simulink model "torqueWalking"  (Simulink 8.8)
settings: Solver=FixedStepDiscrete  StartTime=0.0  StopTime=Config.t_end  FixedStep=Config.t_step  RelTol=1e-3  EnableMultiTasking=on
InitFcn:
  | cd(fileparts(which(bdroot)));
  | initTorqueWalking;
undefined symbols (not defined in the file or in its folder): biasVectorConstraint_feet, Config, ConstraintMatrix_feet, DiscIntNeverNeededParam, Gains, ROBOT_DOF, Sat
libraries: WBToolboxLibrary x98
(part 2 of 3)

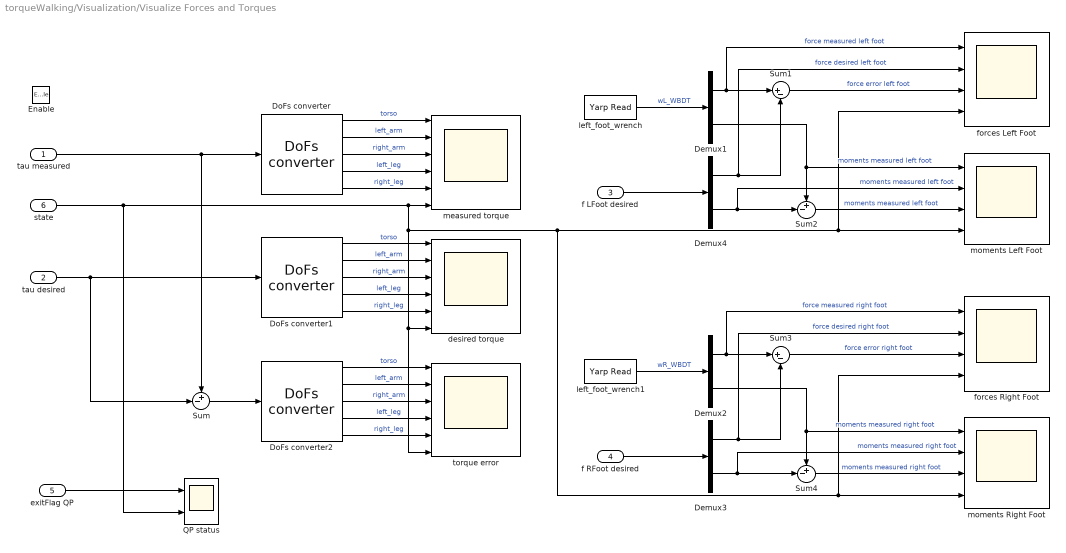
== system torqueWalking/Visualization/Visualize Forces and Torques ==
  tau measured : Inport
  tau desired : Inport  Port=2
  f LFoot desired : Inport  Port=3
  f RFoot desired : Inport  Port=4
  exitFlag QP : Inport  Port=5
  state : Inport  Port=6
  Enable : EnablePort
  Demux{1..4} (4 alike) : Demux  Outputs=[3;3]
  DoFs converter : WBToolboxLibrary/Utilities/DoFs converter  yarp2WBIOption=From WBI to YARP  robotName=WBT_robotName  localName=WBT_modelName  wbiFile=WBT_wbiFilename  wbiList=WBT_wbiList
  DoFs converter1 : WBToolboxLibrary/Utilities/DoFs converter  yarp2WBIOption=From WBI to YARP  robotName=WBT_robotName  localName=WBT_modelName  wbiFile=WBT_wbiFilename  wbiList=WBT_wbiList
  DoFs converter2 : WBToolboxLibrary/Utilities/DoFs converter  yarp2WBIOption=From WBI to YARP  robotName=WBT_robotName  localName=WBT_modelName  wbiFile=WBT_wbiFilename  wbiList=WBT_wbiList
  QP status : Scope  NumInputPorts=2
  Sum : Sum  Inputs=+-|
  Sum1 : Sum  Inputs=|+-
  Sum2 : Sum  Inputs=+-|
  Sum3 : Sum  Inputs=|+-
  Sum4 : Sum  Inputs=+-|
  desired torque : Scope  NumInputPorts=6
  forces Left Foot : Scope  NumInputPorts=4
  forces Right Foot : Scope  NumInputPorts=4
  left_foot_wrench : WBToolboxLibrary/Utilities/Yarp Read  portName=Ports.LEFT_FOOT_EXT_WRENCH  signalSize=6  blocking=off  timestamp=off  autoconnect=on  errorOnConnection=on
  left_foot_wrench1 : WBToolboxLibrary/Utilities/Yarp Read  portName=Ports.LEFT_FOOT_EXT_WRENCH  signalSize=6  blocking=off  timestamp=off  autoconnect=on  errorOnConnection=on
  measured torque : Scope  NumInputPorts=6
  moments Left Foot : Scope  NumInputPorts=4
  moments Right Foot : Scope  NumInputPorts=4
  torque error : Scope  NumInputPorts=6
  wires:
  Sum2/1 -> moments Left Foot/3  "moments measured left foot"
  state/1 -> QP status/2, torque error/6, desired torque/6, forces Right Foot/4, moments Right Foot/4, forces Left Foot/4, moments Left Foot/4, measured torque/6
  DoFs converter1/2 -> desired torque/2  "left_arm"
  Demux4/1 -> forces Left Foot/2, Sum1/2  "force desired left foot"
  DoFs converter2/1 -> torque error/1  "torso"
  DoFs converter1/4 -> desired torque/4  "left_leg"
  Demux4/2 -> moments Left Foot/2, Sum2/2  "moments measured left foot"
  DoFs converter/1 -> measured torque/1  "torso"
  DoFs converter2/3 -> torque error/3  "right_arm"
  f RFoot desired/1 -> Demux3/1
  DoFs converter1/1 -> desired torque/1  "torso"
  Sum4/1 -> moments Right Foot/3  "moments measured right foot"
  tau desired/1 -> Sum/2, DoFs converter1/1
  Demux2/1 -> forces Right Foot/1, Sum3/1  "force measured right foot"
  DoFs converter2/2 -> torque error/2  "left_arm"
  Sum3/1 -> forces Right Foot/3  "force error right foot"
  DoFs converter/5 -> measured torque/5  "right_leg"
  DoFs converter2/5 -> torque error/5  "right_leg"
  exitFlag QP/1 -> QP status/1
  left_foot_wrench/1 -> Demux1/1  "wL_WBDT"
  DoFs converter1/3 -> desired torque/3  "right_arm"
  Demux3/1 -> forces Right Foot/2, Sum3/2  "force desired right foot"
  f LFoot desired/1 -> Demux4/1
  Sum1/1 -> forces Left Foot/3  "force error left foot"
  tau measured/1 -> Sum/1, DoFs converter/1
  DoFs converter1/5 -> desired torque/5  "right_leg"
  DoFs converter/2 -> measured torque/2  "left_arm"
  DoFs converter/3 -> measured torque/3  "right_arm"
  Demux3/2 -> moments Right Foot/2, Sum4/2  "moments measured right foot"
  Sum/1 -> DoFs converter2/1
  Demux1/1 -> forces Left Foot/1, Sum1/1  "force measured left foot"
  DoFs converter/4 -> measured torque/4  "left_leg"
  Demux1/2 -> moments Left Foot/1, Sum2/1  "moments measured left foot"
  left_foot_wrench1/1 -> Demux2/1  "wR_WBDT"
  DoFs converter2/4 -> torque error/4  "left_leg"
  Demux2/2 -> moments Right Foot/1, Sum4/1  "moments measured right foot"

== system torqueWalking/Visualization/Visualize Gain Scheduling ==
  Kp_CoM : Inport
  Kd_CoM : Inport  Port=2
  Kp_LFoot : Inport  Port=3
  Kd_LFoot : Inport  Port=4
  Kp_RFoot : Inport  Port=5
  Kd_RFoot : Inport  Port=6
  Kp_rot_task : Inport  Port=7
  Kd_rot_task : Inport  Port=8
  impedances : Inport  Port=9
  dampings : Inport  Port=10
  state : Inport  Port=11
  Enable : EnablePort
  DoFs converter1 : WBToolboxLibrary/Utilities/DoFs converter  yarp2WBIOption=From WBI to YARP  robotName=WBT_robotName  localName=WBT_modelName  wbiFile=WBT_wbiFilename  wbiList=WBT_wbiList
  DoFs converter4 : WBToolboxLibrary/Utilities/DoFs converter  yarp2WBIOption=From WBI to YARP  robotName=WBT_robotName  localName=WBT_modelName  wbiFile=WBT_wbiFilename  wbiList=WBT_wbiList
  joint position gains : Scope  NumInputPorts=6
  joint valocity gains : Scope  NumInputPorts=6
  pos gains CoM : Scope  NumInputPorts=2
  pos gains LFoot : Scope  NumInputPorts=2
  pos gains RFoot : Scope  NumInputPorts=2
  pos gains rot task : Scope  NumInputPorts=2
  vel gains CoM : Scope  NumInputPorts=2
  vel gains LFoot : Scope  NumInputPorts=2
  vel gains RFoot : Scope  NumInputPorts=2
  vel gains rot task : Scope  NumInputPorts=2
  wires:
  Kp_CoM/1 -> pos gains CoM/1
  Kp_LFoot/1 -> pos gains LFoot/1
  Kp_RFoot/1 -> pos gains RFoot/1
  Kp_rot_task/1 -> pos gains rot task/1
  state/1 -> vel gains LFoot/2, pos gains LFoot/2, vel gains CoM/2, vel gains rot task/2, pos gains rot task/2, vel gains RFoot/2, joint valocity gains/6, joint position gains/6, pos gains RFoot/2, pos gains CoM/2
  Kd_CoM/1 -> vel gains CoM/1
  Kd_LFoot/1 -> vel gains LFoot/1
  Kd_RFoot/1 -> vel gains RFoot/1
  Kd_rot_task/1 -> vel gains rot task/1
  DoFs converter4/2 -> joint position gains/2  "left_arm"
  DoFs converter4/1 -> joint position gains/1  "torso"
  DoFs converter4/4 -> joint position gains/4  "left_leg"
  DoFs converter4/3 -> joint position gains/3  "right_arm"
  DoFs converter4/5 -> joint position gains/5  "right_leg"
  DoFs converter1/2 -> joint valocity gains/2  "left_arm"
  DoFs converter1/1 -> joint valocity gains/1  "torso"
  DoFs converter1/4 -> joint valocity gains/4  "left_leg"
  DoFs converter1/3 -> joint valocity gains/3  "right_arm"
  DoFs converter1/5 -> joint valocity gains/5  "right_leg"
  impedances/1 -> DoFs converter4/1
  dampings/1 -> DoFs converter1/1

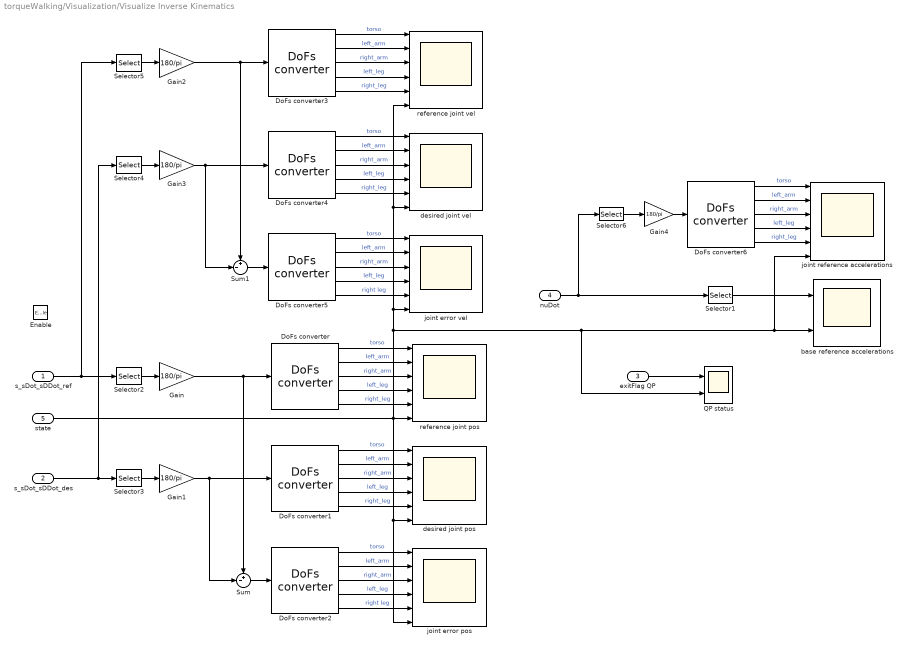
== system torqueWalking/Visualization/Visualize Inverse Kinematics ==
  s_sDot_sDDot_ref : Inport
  s_sDot_sDDot_des : Inport  Port=2
  exitFlag QP : Inport  Port=3
  nuDot : Inport  Port=4
  state : Inport  Port=5
  Enable : EnablePort
  DoFs converter{,1..6} (7 alike) : WBToolboxLibrary/Utilities/DoFs converter  yarp2WBIOption=From WBI to YARP  robotName=WBT_robotName  localName=WBT_modelName  wbiFile=WBT_wbiFilename  wbiList=WBT_wbiList
  Gain{,1..4} (5 alike) : Gain  Gain=180/pi
  QP status : Scope  NumInputPorts=2
  Selector1 : Selector  InputPortWidth=ROBOT_DOF+6  IndexOptions=Index vector (dialog)  Indices=[1:6]  OutputSizes=1
  Selector2 : Selector  NumberOfDimensions=2  InputPortWidth=ROBOT_DOF  IndexOptions=Index vector (dialog),Index vector (dialog)  Indices=[1:ROBOT_DOF],1  OutputSizes=1,1
  Selector3 : Selector  NumberOfDimensions=2  InputPortWidth=ROBOT_DOF  IndexOptions=Index vector (dialog),Index vector (dialog)  Indices=[1:ROBOT_DOF],1  OutputSizes=1,1
  Selector4 : Selector  NumberOfDimensions=2  InputPortWidth=ROBOT_DOF  IndexOptions=Index vector (dialog),Index vector (dialog)  Indices=[1:ROBOT_DOF],2  OutputSizes=1,1
  Selector5 : Selector  NumberOfDimensions=2  InputPortWidth=ROBOT_DOF  IndexOptions=Index vector (dialog),Index vector (dialog)  Indices=[1:ROBOT_DOF],2  OutputSizes=1,1
  Selector6 : Selector  InputPortWidth=ROBOT_DOF+6  IndexOptions=Index vector (dialog)  Indices=[7:ROBOT_DOF+6]  OutputSizes=1
  Sum : Sum  Inputs=+-|
  Sum1 : Sum  Inputs=+-|
  base reference accelerations : Scope  NumInputPorts=2
  desired joint pos : Scope  NumInputPorts=6
  desired joint vel : Scope  NumInputPorts=6
  joint error pos : Scope  NumInputPorts=6
  joint error vel : Scope  NumInputPorts=6
  joint reference accelerations : Scope  NumInputPorts=6
  reference joint pos : Scope  NumInputPorts=6
  reference joint vel : Scope  NumInputPorts=6
  wires:
  DoFs converter1/2 -> desired joint pos/2  "left_arm"
  DoFs converter/5 -> reference joint pos/5  "right_leg"
  DoFs converter2/1 -> joint error pos/1  "torso"
  DoFs converter/4 -> reference joint pos/4  "left_leg"
  DoFs converter/2 -> reference joint pos/2  "left_arm"
  DoFs converter1/1 -> desired joint pos/1  "torso"
  DoFs converter1/4 -> desired joint pos/4  "left_leg"
  DoFs converter1/3 -> desired joint pos/3  "right_arm"
  DoFs converter/3 -> reference joint pos/3  "right_arm"
  DoFs converter2/2 -> joint error pos/2  "left_arm"
  DoFs converter/1 -> reference joint pos/1  "torso"
  DoFs converter1/5 -> desired joint pos/5  "right_leg"
  DoFs converter2/4 -> joint error pos/4  "left_leg"
  Sum/1 -> DoFs converter2/1
  DoFs converter2/3 -> joint error pos/3  "right_arm"
  Gain/1 -> Sum/1, DoFs converter/1
  Gain1/1 -> Sum/2, DoFs converter1/1
  DoFs converter4/2 -> desired joint vel/2  "left_arm"
  DoFs converter3/5 -> reference joint vel/5  "right_leg"
  DoFs converter5/1 -> joint error vel/1  "torso"
  DoFs converter3/4 -> reference joint vel/4  "left_leg"
  DoFs converter3/2 -> reference joint vel/2  "left_arm"
  s_sDot_sDDot_ref/1 -> Selector5/1, Selector2/1
  DoFs converter4/1 -> desired joint vel/1  "torso"
  DoFs converter4/4 -> desired joint vel/4  "left_leg"
  DoFs converter4/3 -> desired joint vel/3  "right_arm"
  DoFs converter3/3 -> reference joint vel/3  "right_arm"
  DoFs converter5/2 -> joint error vel/2  "left_arm"
  DoFs converter3/1 -> reference joint vel/1  "torso"
  s_sDot_sDDot_des/1 -> Selector4/1, Selector3/1
  DoFs converter4/5 -> desired joint vel/5  "right_leg"
  DoFs converter5/4 -> joint error vel/4  "left_leg"
  Sum1/1 -> DoFs converter5/1
  DoFs converter5/3 -> joint error vel/3  "right_arm"
  Gain2/1 -> Sum1/1, DoFs converter3/1
  Gain3/1 -> Sum1/2, DoFs converter4/1
  DoFs converter5/5 -> joint error vel/5  "right leg"
  DoFs converter2/5 -> joint error pos/5  "right leg"
  Selector1/1 -> base reference accelerations/1
  Selector2/1 -> Gain/1
  Selector3/1 -> Gain1/1
  Selector4/1 -> Gain3/1
  Selector5/1 -> Gain2/1
  DoFs converter6/5 -> joint reference accelerations/5  "right_leg"
  DoFs converter6/1 -> joint reference accelerations/1  "torso"
  DoFs converter6/4 -> joint reference accelerations/4  "left_leg"
  DoFs converter6/3 -> joint reference accelerations/3  "right_arm"
  DoFs converter6/2 -> joint reference accelerations/2  "left_arm"
  nuDot/1 -> Selector6/1, Selector1/1
  Gain4/1 -> DoFs converter6/1
  Selector6/1 -> Gain4/1
  state/1 -> reference joint vel/6, desired joint vel/6, joint error vel/6, QP status/2, joint reference accelerations/6, base reference accelerations/2, joint error pos/6, desired joint pos/6, reference joint pos/6
  exitFlag QP/1 -> QP status/1

== system torqueWalking/Visualization/Visualize Robot State ==
  s : Inport
  w_H_b : Inport  Port=2
  nu : Inport  Port=3
  state : Inport  Port=4
  s_des : Inport  Port=5
  feetInContact : Inport  Port=6
  Enable : EnablePort
  DoFs converter{,1..3} (4 alike) : WBToolboxLibrary/Utilities/DoFs converter  yarp2WBIOption=From WBI to YARP  robotName=WBT_robotName  localName=WBT_modelName  wbiFile=WBT_wbiFilename  wbiList=WBT_wbiList
  Gain : Gain  Gain=180/pi
  Gain1 : Gain  Gain=180/pi
  Gain2 : Gain  Gain=180/pi
  Selector : Selector  NumberOfDimensions=2  InputPortWidth=3  IndexOptions=Index vector (dialog),Index vector (dialog)  Indices=[1:3],4  OutputSizes=1,1
  Selector1 : Selector  InputPortWidth=ROBOT_DOF+6  IndexOptions=Index vector (dialog)  Indices=[1:6]  OutputSizes=1
  Selector2 : Selector  InputPortWidth=ROBOT_DOF+6  IndexOptions=Index vector (dialog)  Indices=[7:ROBOT_DOF+6]  OutputSizes=1
  Sum : Sum  Inputs=+-|
  base position : Scope  NumInputPorts=2
  base velocity : Scope  NumInputPorts=2
  desired joint pos : Scope  NumInputPorts=6
  feet in contact : Scope  NumInputPorts=2
  joint error : Scope  NumInputPorts=6
  joint velocity : Scope  NumInputPorts=6
  measured joint pos : Scope  NumInputPorts=6
  wires:
  DoFs converter1/2 -> desired joint pos/2  "left_arm"
  DoFs converter/5 -> measured joint pos/5  "right_leg"
  DoFs converter2/1 -> joint error/1  "torso"
  DoFs converter/4 -> measured joint pos/4  "left_leg"
  DoFs converter/2 -> measured joint pos/2  "left_arm"
  s/1 -> Gain/1
  DoFs converter1/1 -> desired joint pos/1  "torso"
  DoFs converter1/4 -> desired joint pos/4  "left_leg"
  DoFs converter1/3 -> desired joint pos/3  "right_arm"
  DoFs converter/3 -> measured joint pos/3  "right_arm"
  DoFs converter2/5 -> joint error/5  "right_leg"
  DoFs converter2/2 -> joint error/2  "left_arm"
  DoFs converter/1 -> measured joint pos/1  "torso"
  s_des/1 -> Gain1/1
  DoFs converter1/5 -> desired joint pos/5  "right_leg"
  DoFs converter2/4 -> joint error/4  "left_leg"
  Sum/1 -> DoFs converter2/1
  DoFs converter2/3 -> joint error/3  "right_arm"
  DoFs converter3/5 -> joint velocity/5  "right_leg"
  DoFs converter3/1 -> joint velocity/1  "torso"
  DoFs converter3/4 -> joint velocity/4  "left_leg"
  DoFs converter3/3 -> joint velocity/3  "right_arm"
  DoFs converter3/2 -> joint velocity/2  "left_arm"
  nu/1 -> Selector2/1, Selector1/1
  w_H_b/1 -> Selector/1
  Gain/1 -> Sum/1, DoFs converter/1
  Gain1/1 -> Sum/2, DoFs converter1/1
  Gain2/1 -> DoFs converter3/1
  Selector/1 -> base position/1
  Selector2/1 -> Gain2/1
  state/1 -> measured joint pos/6, joint velocity/6, base velocity/2, feet in contact/2, base position/2, joint error/6, desired joint pos/6
  Selector1/1 -> base velocity/1
  feetInContact/1 -> feet in contact/1

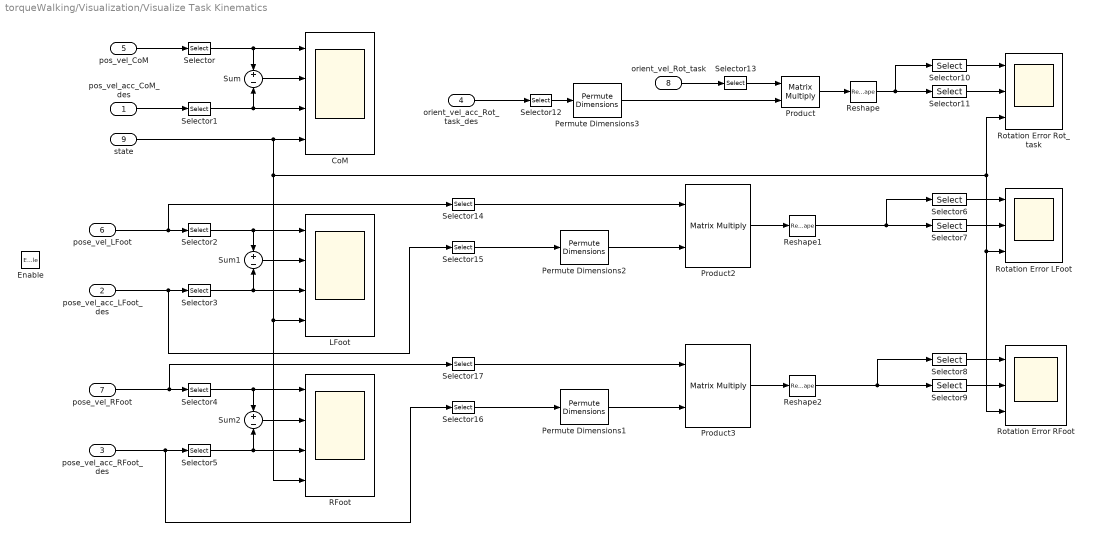
== system torqueWalking/Visualization/Visualize Task Kinematics ==
  pos_vel_acc_CoM_des : Inport
  pose_vel_acc_LFoot_des : Inport  Port=2
  pose_vel_acc_RFoot_des : Inport  Port=3
  orient_vel_acc_Rot_task_des : Inport  Port=4
  pos_vel_CoM : Inport  Port=5
  pose_vel_LFoot : Inport  Port=6
  pose_vel_RFoot : Inport  Port=7
  orient_vel_Rot_task : Inport  Port=8
  state : Inport  Port=9
  Enable : EnablePort
  CoM : Scope  NumInputPorts=4
  LFoot : Scope  NumInputPorts=4
  Permute Dimensions1 : PermuteDimensions
  Permute Dimensions2 : PermuteDimensions
  Permute Dimensions3 : PermuteDimensions
  Product : Product  Multiplication=Matrix(*)
  Product2 : Product  Multiplication=Matrix(*)
  Product3 : Product  Multiplication=Matrix(*)
  RFoot : Scope  NumInputPorts=4
  Reshape : Reshape
  Reshape1 : Reshape
  Reshape2 : Reshape
  Rotation Error LFoot : Scope  NumInputPorts=3
  Rotation Error RFoot : Scope  NumInputPorts=3
  Rotation Error Rot_task : Scope  NumInputPorts=3
  Selector{,1..5} (6 alike) : Selector  NumberOfDimensions=2  InputPortWidth=3  IndexOptions=Index vector (dialog),Index vector (dialog)  Indices=[1:3],1  OutputSizes=1,1
  Selector10 : Selector  InputPortWidth=9  IndexOptions=Index vector (dialog)  Indices=[1 5 9]  OutputSizes=1
  Selector11 : Selector  InputPortWidth=9  IndexOptions=Index vector (dialog)  Indices=[2 3 4 6 7 8]  OutputSizes=1
  Selector12 : Selector  NumberOfDimensions=2  InputPortWidth=3  IndexOptions=Index vector (dialog),Index vector (dialog)  Indices=[1:3],[1:3]  OutputSizes=1,1
  Selector13 : Selector  NumberOfDimensions=2  InputPortWidth=3  IndexOptions=Index vector (dialog),Index vector (dialog)  Indices=[1:3],[1:3]  OutputSizes=1,1
  Selector{14..17} (4 alike) : Selector  NumberOfDimensions=2  InputPortWidth=3  IndexOptions=Index vector (dialog),Index vector (dialog)  Indices=[4:6],[1:3]  OutputSizes=1,1
  Selector6 : Selector  InputPortWidth=9  IndexOptions=Index vector (dialog)  Indices=[1 5 9]  OutputSizes=1
  Selector7 : Selector  InputPortWidth=9  IndexOptions=Index vector (dialog)  Indices=[2 3 4 6 7 8]  OutputSizes=1
  Selector8 : Selector  InputPortWidth=9  IndexOptions=Index vector (dialog)  Indices=[1 5 9]  OutputSizes=1
  Selector9 : Selector  InputPortWidth=9  IndexOptions=Index vector (dialog)  Indices=[2 3 4 6 7 8]  OutputSizes=1
  Sum : Sum  Inputs=+|-
  Sum1 : Sum  Inputs=+|-
  Sum2 : Sum  Inputs=+|-
  wires:
  Selector1/1 -> CoM/3, Sum/2
  Sum/1 -> CoM/2
  pos_vel_CoM/1 -> Selector/1
  pos_vel_acc_CoM_des/1 -> Selector1/1
  Selector2/1 -> LFoot/1, Sum1/1
  Selector3/1 -> LFoot/3, Sum1/2
  Sum1/1 -> LFoot/2
  Selector4/1 -> RFoot/1, Sum2/1
  Selector5/1 -> RFoot/3, Sum2/2
  Sum2/1 -> RFoot/2
  pose_vel_RFoot/1 -> Selector17/1, Selector4/1
  state/1 -> RFoot/4, LFoot/4, Rotation Error RFoot/3, Rotation Error LFoot/3, Rotation Error Rot_task/3, CoM/4
  pose_vel_acc_RFoot_des/1 -> Selector5/1, Selector16/1
  Permute Dimensions2/1 -> Product2/2
  Permute Dimensions1/1 -> Product3/2
  Permute Dimensions3/1 -> Product/2
  Product2/1 -> Reshape1/1
  Product3/1 -> Reshape2/1
  Product/1 -> Reshape/1
  Selector13/1 -> Product/1
  pose_vel_LFoot/1 -> Selector14/1, Selector2/1
  Reshape1/1 -> Selector6/1, Selector7/1
  Reshape2/1 -> Selector8/1, Selector9/1
  Reshape/1 -> Selector10/1, Selector11/1
  Selector7/1 -> Rotation Error LFoot/2
  Selector6/1 -> Rotation Error LFoot/1
  Selector8/1 -> Rotation Error RFoot/1
  Selector9/1 -> Rotation Error RFoot/2
  Selector10/1 -> Rotation Error Rot_task/1
  Selector11/1 -> Rotation Error Rot_task/2
  Selector12/1 -> Permute Dimensions3/1
  pose_vel_acc_LFoot_des/1 -> Selector15/1, Selector3/1
  orient_vel_acc_Rot_task_des/1 -> Selector12/1
  orient_vel_Rot_task/1 -> Selector13/1
  Selector14/1 -> Product2/1
  Selector15/1 -> Permute Dimensions2/1
  Selector16/1 -> Permute Dimensions1/1
  Selector17/1 -> Product3/1
  Selector/1 -> Sum/1, CoM/1

== system torqueWalking/synchronizer/GAZEBO_SYNCHRONIZER ==
  Enable : EnablePort
  Simulator Synchronizer : WBToolboxLibrary/Utilities/Simulator Synchronizer  period=Config.t_step  serverPortName='/clock/rpc'  clientPortName='/WBT_synchronizer/rpc:o'

== system torqueWalking/synchronizer/REAL_TIME_SYNC ==
  Enable : EnablePort
  Real Time Synchronizer : WBToolboxLibrary/Utilities/Real Time Synchronizer  period=Config.t_step

== system torqueWalking/Dynamics and Kinematics/Compute Dynamic and Kinematic Quantities/Jacobians and JDot_nu ==
  s : Inport
  nu_b : Inport  Port=2
  sDot : Inport  Port=3
  w_H_b : Inport  Port=4
  DotJ Nu CoM : WBToolboxLibrary/wholeBodyModel/Jacobians/DotJ Nu  frameName=Frames.COM  robotName=WBT_robotName  localName=WBT_modelName  wbiFile=WBT_wbiFilename  wbiList=WBT_wbiList
  DotJ Nu LFoot : WBToolboxLibrary/wholeBodyModel/Jacobians/DotJ Nu  frameName=Frames.LEFT_FOOT  robotName=WBT_robotName  localName=WBT_modelName  wbiFile=WBT_wbiFilename  wbiList=WBT_wbiList
  DotJ Nu RFoot : WBToolboxLibrary/wholeBodyModel/Jacobians/DotJ Nu  frameName=Frames.RIGHT_FOOT  robotName=WBT_robotName  localName=WBT_modelName  wbiFile=WBT_wbiFilename  wbiList=WBT_wbiList
  DotJ Nu rotational task : WBToolboxLibrary/wholeBodyModel/Jacobians/DotJ Nu  frameName=Frames.ROT_TASK_LINK  robotName=WBT_robotName  localName=WBT_modelName  wbiFile=WBT_wbiFilename  wbiList=WBT_wbiList
  Jacobian CoM : WBToolboxLibrary/wholeBodyModel/Jacobians/Jacobian  frameName=Frames.COM  robotName=WBT_robotName  localName=WBT_modelName  wbiFile=WBT_wbiFilename  wbiList=WBT_wbiList
  Jacobian LFoot : WBToolboxLibrary/wholeBodyModel/Jacobians/Jacobian  frameName=Frames.LEFT_FOOT  robotName=WBT_robotName  localName=WBT_modelName  wbiFile=WBT_wbiFilename  wbiList=WBT_wbiList
  Jacobian RFoot : WBToolboxLibrary/wholeBodyModel/Jacobians/Jacobian  frameName=Frames.RIGHT_FOOT  robotName=WBT_robotName  localName=WBT_modelName  wbiFile=WBT_wbiFilename  wbiList=WBT_wbiList
  Jacobian rotational task : WBToolboxLibrary/wholeBodyModel/Jacobians/Jacobian  frameName=Frames.ROT_TASK_LINK  robotName=WBT_robotName  localName=WBT_modelName  wbiFile=WBT_wbiFilename  wbiList=WBT_wbiList
  J_LFoot : Outport
  J_RFoot : Outport  Port=2
  J_CoM : Outport  Port=3
  J_rot_task : Outport  Port=4
  JDot_nu_LFoot : Outport  Port=5
  JDot_nu_RFoot : Outport  Port=6
  JDot_nu_CoM : Outport  Port=7
  JDot_nu_rot_task : Outport  Port=8
  wires:
  Jacobian CoM/1 -> J_CoM/1
  Jacobian rotational task/1 -> J_rot_task/1
  Jacobian LFoot/1 -> J_LFoot/1
  Jacobian RFoot/1 -> J_RFoot/1
  w_H_b/1 -> Jacobian RFoot/1, Jacobian LFoot/1, DotJ Nu RFoot/1, DotJ Nu LFoot/1, DotJ Nu rotational task/1, DotJ Nu CoM/1, Jacobian CoM/1, Jacobian rotational task/1
  sDot/1 -> DotJ Nu RFoot/4, DotJ Nu LFoot/4, DotJ Nu rotational task/4, DotJ Nu CoM/4
  nu_b/1 -> DotJ Nu CoM/3, DotJ Nu RFoot/3, DotJ Nu LFoot/3, DotJ Nu rotational task/3
  s/1 -> DotJ Nu RFoot/2, DotJ Nu LFoot/2, DotJ Nu rotational task/2, DotJ Nu CoM/2, Jacobian RFoot/2, Jacobian CoM/2, Jacobian rotational task/2, Jacobian LFoot/2
  DotJ Nu RFoot/1 -> JDot_nu_RFoot/1
  DotJ Nu LFoot/1 -> JDot_nu_LFoot/1
  DotJ Nu rotational task/1 -> JDot_nu_rot_task/1
  DotJ Nu CoM/1 -> JDot_nu_CoM/1

== system torqueWalking/Dynamics and Kinematics/Compute Dynamic and Kinematic Quantities/Mass Matrix and Bias Forces ==
  s : Inport
  nu_b : Inport  Port=2
  sDot : Inport  Port=3
  w_H_b : Inport  Port=4
  Get Bias Forces : WBToolboxLibrary/wholeBodyModel/Dynamics/Get Bias Forces  robotName=WBT_robotName  localName=WBT_modelName  wbiFile=WBT_wbiFilename  wbiList=WBT_wbiList  explicitGravity=off
  Mass Matrix : WBToolboxLibrary/wholeBodyModel/Dynamics/Mass Matrix  robotName=WBT_robotName  localName=WBT_modelName  wbiFile=WBT_wbiFilename  wbiList=WBT_wbiList
  h(q,nu) : Outport
  M(q) : Outport  Port=2
  wires:
  w_H_b/1 -> Mass Matrix/1, Get Bias Forces/1
  s/1 -> Mass Matrix/2, Get Bias Forces/2
  sDot/1 -> Get Bias Forces/4
  nu_b/1 -> Get Bias Forces/3
  Get Bias Forces/1 -> h(q,nu)/1
  Mass Matrix/1 -> M(q)/1

== system torqueWalking/Dynamics and Kinematics/Initial Conditions/Compute world to base transform ==
  s : Inport
  Constant : Constant  Value=Config.LFoot_in_contact_at0
  Constant6 : Constant  Value=eye(4)
  "Inv\\*  " : Product  Inputs=/*  Multiplication=Matrix(*)
  Switch6 : Switch  Criteria=u2 > Threshold
  left foot : WBToolboxLibrary/wholeBodyModel/Kinematics/Forward Kinematics  frameName=Frames.LEFT_FOOT  robotName=WBT_robotName  localName=WBT_modelName  wbiFile=WBT_wbiFilename  wbiList=WBT_wbiList
  left foot1 : WBToolboxLibrary/wholeBodyModel/Kinematics/Forward Kinematics  frameName=Frames.RIGHT_FOOT  robotName=WBT_robotName  localName=WBT_modelName  wbiFile=WBT_wbiFilename  wbiList=WBT_wbiList
  root_link : WBToolboxLibrary/wholeBodyModel/Kinematics/Forward Kinematics  frameName='root_link'  robotName=WBT_robotName  localName=WBT_modelName  wbiFile=WBT_wbiFilename  wbiList=WBT_wbiList
  w_H_b : Outport
  wires:
  Constant/1 -> Switch6/2
  left foot1/1 -> Switch6/1
  s/1 -> root_link/2, left foot/2, left foot1/2
  left foot/1 -> Switch6/3
  "Inv\\*  "/1 -> w_H_b/1
  Constant6/1 -> left foot/1, root_link/1, left foot1/1
  Switch6/1 -> "Inv\\*  "/1
  root_link/1 -> "Inv\\*  "/2

== system torqueWalking/Dynamics and Kinematics/Initial Conditions/compute state velocity ==
  s : Inport
  w_H_b : Inport  Port=2
  "feetInContact " : Inport  Port=3
  sDot : Inport  Port=4
  Compute Base Velocity : MATLAB Function  TreatAsAtomicUnit=on
  Feet Jacobians : Subsystem
  Mux : Mux  Inputs=2
  nu : Outport
  wires:
  w_H_b/1 -> Feet Jacobians/2(w_H_b)
  "feetInContact "/1 -> Compute Base Velocity/3(feetInContact)
  Mux/1 -> nu/1
  s/1 -> Feet Jacobians/1(s)
  Compute Base Velocity/1(nu_b) -> Mux/1
  sDot/1 -> Mux/2, Compute Base Velocity/4(sDot)
  Feet Jacobians/1(J_LFoot) -> Compute Base Velocity/1(J_LeftFoot)
  Feet Jacobians/2(J_RFoot) -> Compute Base Velocity/2(J_RightFoot)

== system torqueWalking/Dynamics and Kinematics/Inverse Kinematics/ComputeTasksPoseAndVelocity ==
  J_LFoot : Inport
  J_RFoot : Inport  Port=2
  J_CoM : Inport  Port=3
  J_rot_task : Inport  Port=4
  qj : Inport  Port=5
  w_H_b : Inport  Port=6
  nu : Inport  Port=7
  Compose Task Pose and Velocity : MATLAB Function  TreatAsAtomicUnit=on
  Product{,1..3} (4 alike) : Product  Multiplication=Matrix(*)
  Task position and orientation : Subsystem
  pos_vel_CoM : Outport
  pose_vel_LFoot : Outport  Port=2
  pose_vel_RFoot : Outport  Port=3
  orient_vel_rot_task : Outport  Port=4
  wires:
  Compose Task Pose and Velocity/3(pose_vel_RFoot) -> pose_vel_RFoot/1
  Compose Task Pose and Velocity/2(pose_vel_LFoot) -> pose_vel_LFoot/1
  Compose Task Pose and Velocity/1(pos_vel_CoM) -> pos_vel_CoM/1
  Compose Task Pose and Velocity/4(orient_vel_rot_task) -> orient_vel_rot_task/1
  nu/1 -> Product1/2, Product/2, Product2/2, Product3/2
  J_rot_task/1 -> Product3/1
  Product/1 -> Compose Task Pose and Velocity/1(vel_CoM)
  Product1/1 -> Compose Task Pose and Velocity/2(vel_LFoot)
  Product2/1 -> Compose Task Pose and Velocity/3(vel_RFoot)
  Product3/1 -> Compose Task Pose and Velocity/4(vel_rot_task)
  qj/1 -> Task position and orientation/1(s)
  w_H_b/1 -> Task position and orientation/2(w_H_b)
  Task position and orientation/1(w_H_CoM) -> Compose Task Pose and Velocity/5(w_H_CoM)
  Task position and orientation/2(w_H_l_sole) -> Compose Task Pose and Velocity/6(w_H_l_sole)
  Task position and orientation/3(w_H_r_sole) -> Compose Task Pose and Velocity/7(w_H_r_sole)
  Task position and orientation/4(w_H_rot_task) -> Compose Task Pose and Velocity/8(w_H_rot_task)
  J_LFoot/1 -> Product1/1
  J_CoM/1 -> Product/1
  J_RFoot/1 -> Product2/1

== system torqueWalking/Dynamics and Kinematics/Inverse Kinematics/Jacobians and JDot_nu ==
  s : Inport
  w_H_b : Inport  Port=2
  nu_b : Inport  Port=3
  sDot : Inport  Port=4
  DotJ Nu CoM : WBToolboxLibrary/wholeBodyModel/Jacobians/DotJ Nu  frameName=Frames.COM  robotName=WBT_robotName  localName=WBT_modelName  wbiFile=WBT_wbiFilename  wbiList=WBT_wbiList
  DotJ Nu LFoot : WBToolboxLibrary/wholeBodyModel/Jacobians/DotJ Nu  frameName=Frames.LEFT_FOOT  robotName=WBT_robotName  localName=WBT_modelName  wbiFile=WBT_wbiFilename  wbiList=WBT_wbiList
  DotJ Nu Rfoot : WBToolboxLibrary/wholeBodyModel/Jacobians/DotJ Nu  frameName=Frames.RIGHT_FOOT  robotName=WBT_robotName  localName=WBT_modelName  wbiFile=WBT_wbiFilename  wbiList=WBT_wbiList
  DotJ Nu rotational task : WBToolboxLibrary/wholeBodyModel/Jacobians/DotJ Nu  frameName=Frames.ROT_TASK_LINK  robotName=WBT_robotName  localName=WBT_modelName  wbiFile=WBT_wbiFilename  wbiList=WBT_wbiList
  Jacobian CoM : WBToolboxLibrary/wholeBodyModel/Jacobians/Jacobian  frameName=Frames.COM  robotName=WBT_robotName  localName=WBT_modelName  wbiFile=WBT_wbiFilename  wbiList=WBT_wbiList
  Jacobian LFoot : WBToolboxLibrary/wholeBodyModel/Jacobians/Jacobian  frameName=Frames.LEFT_FOOT  robotName=WBT_robotName  localName=WBT_modelName  wbiFile=WBT_wbiFilename  wbiList=WBT_wbiList
  Jacobian RFoot : WBToolboxLibrary/wholeBodyModel/Jacobians/Jacobian  frameName=Frames.RIGHT_FOOT  robotName=WBT_robotName  localName=WBT_modelName  wbiFile=WBT_wbiFilename  wbiList=WBT_wbiList
  Jacobian rotational task : WBToolboxLibrary/wholeBodyModel/Jacobians/Jacobian  frameName=Frames.ROT_TASK_LINK  robotName=WBT_robotName  localName=WBT_modelName  wbiFile=WBT_wbiFilename  wbiList=WBT_wbiList
  J_LFoot : Outport
  J_RFoot : Outport  Port=2
  J_CoM : Outport  Port=3
  J_rot_task : Outport  Port=4
  JDot_nu_LFoot : Outport  Port=5
  JDot_nu_RFoot : Outport  Port=6
  JDot_nu_CoM : Outport  Port=7
  JDot_nu_rot_task : Outport  Port=8
  wires:
  Jacobian CoM/1 -> J_CoM/1
  Jacobian rotational task/1 -> J_rot_task/1
  Jacobian LFoot/1 -> J_LFoot/1
  Jacobian RFoot/1 -> J_RFoot/1
  w_H_b/1 -> Jacobian RFoot/1, Jacobian LFoot/1, DotJ Nu Rfoot/1, DotJ Nu LFoot/1, DotJ Nu rotational task/1, DotJ Nu CoM/1, Jacobian CoM/1, Jacobian rotational task/1
  sDot/1 -> DotJ Nu Rfoot/4, DotJ Nu LFoot/4, DotJ Nu rotational task/4, DotJ Nu CoM/4
  nu_b/1 -> DotJ Nu CoM/3, DotJ Nu Rfoot/3, DotJ Nu LFoot/3, DotJ Nu rotational task/3
  s/1 -> DotJ Nu Rfoot/2, DotJ Nu LFoot/2, DotJ Nu rotational task/2, DotJ Nu CoM/2, Jacobian RFoot/2, Jacobian CoM/2, Jacobian rotational task/2, Jacobian LFoot/2
  DotJ Nu Rfoot/1 -> JDot_nu_RFoot/1
  DotJ Nu LFoot/1 -> JDot_nu_LFoot/1
  DotJ Nu rotational task/1 -> JDot_nu_rot_task/1
  DotJ Nu CoM/1 -> JDot_nu_CoM/1

== system torqueWalking/Dynamics and Kinematics/Inverse Kinematics/QP-Based Inverse Kinematics ==
  q_0 : Inport
  nu_0 : Inport  Port=2
  s_sDot_sDDot_ref : Inport  Port=3
  J : Inport  Port=4
  JDot_nu : Inport  Port=5
  acc_task_star : Inport  Port=6
  impedances : Inport  Port=7
  dampings : Inport  Port=8
  "Compute QP Hessian, gradient and constraints " : MATLAB Function  TreatAsAtomicUnit=on
  QP Solver (inverse kinematics) : Subsystem
  Selector3 : Selector  InputPortWidth=ROBOT_DOF+16  IndexOptions=Index vector (dialog)  Indices=[17:ROBOT_DOF+16]  OutputSizes=1
  inverse kinematics integration : Subsystem
  s_sDot_sDDot_des : Outport
  ExitFlagQP : Outport  Port=2
  nuDot : Outport  Port=3
  q : Outport  Port=4
  nu : Outport  Port=5
  wires:
  q_0/1 -> inverse kinematics integration/3(q_0)
  nu_0/1 -> inverse kinematics integration/2(nu_0)
  QP Solver (inverse kinematics)/1(nuDot) -> inverse kinematics integration/1(nuDot), nuDot/1
  "Compute QP Hessian, gradient and constraints "/4(biasVectorConstraint) -> QP Solver (inverse kinematics)/4(biasVectorConstraint)
  "Compute QP Hessian, gradient and constraints "/3(ConstraintMatrix) -> QP Solver (inverse kinematics)/3(ConstraintMatrix)
  "Compute QP Hessian, gradient and constraints "/2(gradient) -> QP Solver (inverse kinematics)/2(gradient)
  "Compute QP Hessian, gradient and constraints "/1(Hessian) -> QP Solver (inverse kinematics)/1(Hessian)
  acc_task_star/1 -> "Compute QP Hessian, gradient and constraints "/8(acc_task_star)
  JDot_nu/1 -> "Compute QP Hessian, gradient and constraints "/7(JDot_nu)
  impedances/1 -> "Compute QP Hessian, gradient and constraints "/4(impedances)
  dampings/1 -> "Compute QP Hessian, gradient and constraints "/5(dampings)
  s_sDot_sDDot_ref/1 -> "Compute QP Hessian, gradient and constraints "/3(s_sDot_sDDot_ref)
  inverse kinematics integration/3(s_sDot_sDDot_des) -> s_sDot_sDDot_des/1
  inverse kinematics integration/2(q) -> q/1, Selector3/1
  Selector3/1 -> "Compute QP Hessian, gradient and constraints "/1(s)
  QP Solver (inverse kinematics)/2(ExitFlagQP) -> ExitFlagQP/1
  J/1 -> "Compute QP Hessian, gradient and constraints "/6(J)
  inverse kinematics integration/1(nu) -> nu/1, "Compute QP Hessian, gradient and constraints "/2(nu)

== system torqueWalking/Dynamics and Kinematics/Task Accelerations/ComputeTasksPoseAndVelocity ==
  J_LFoot : Inport
  J_RFoot : Inport  Port=2
  J_CoM : Inport  Port=3
  J_rot_task : Inport  Port=4
  s : Inport  Port=5
  w_H_b : Inport  Port=6
  nu : Inport  Port=7
  Compose Task Pose and Velocity : MATLAB Function  TreatAsAtomicUnit=on
  Product{,1..3} (4 alike) : Product  Multiplication=Matrix(*)
  Task position and orientation : Subsystem
  pos_vel_CoM : Outport
  pose_vel_LFoot : Outport  Port=2
  pose_vel_RFoot : Outport  Port=3
  orient_vel_rot_task : Outport  Port=4
  w_H_l_sole : Outport  Port=5
  w_H_r_sole : Outport  Port=6
  wires:
  Compose Task Pose and Velocity/3(pose_vel_RFoot) -> pose_vel_RFoot/1
  Compose Task Pose and Velocity/2(pose_vel_LFoot) -> pose_vel_LFoot/1
  Compose Task Pose and Velocity/1(pos_vel_CoM) -> pos_vel_CoM/1
  Compose Task Pose and Velocity/4(orient_vel_rot_task) -> orient_vel_rot_task/1
  nu/1 -> Product1/2, Product/2, Product2/2, Product3/2
  J_rot_task/1 -> Product3/1
  Product/1 -> Compose Task Pose and Velocity/1(vel_CoM)
  Product1/1 -> Compose Task Pose and Velocity/2(vel_LFoot)
  Product2/1 -> Compose Task Pose and Velocity/3(vel_RFoot)
  Product3/1 -> Compose Task Pose and Velocity/4(vel_rot_task)
  s/1 -> Task position and orientation/1(s)
  w_H_b/1 -> Task position and orientation/2(w_H_b)
  Task position and orientation/1(w_H_CoM) -> Compose Task Pose and Velocity/5(w_H_CoM)
  Task position and orientation/2(w_H_l_sole) -> w_H_l_sole/1, Compose Task Pose and Velocity/6(w_H_l_sole)
  Task position and orientation/3(w_H_r_sole) -> w_H_r_sole/1, Compose Task Pose and Velocity/7(w_H_r_sole)
  Task position and orientation/4(w_H_rot_task) -> Compose Task Pose and Velocity/8(w_H_rot_task)
  J_RFoot/1 -> Product2/1
  J_LFoot/1 -> Product1/1
  J_CoM/1 -> Product/1

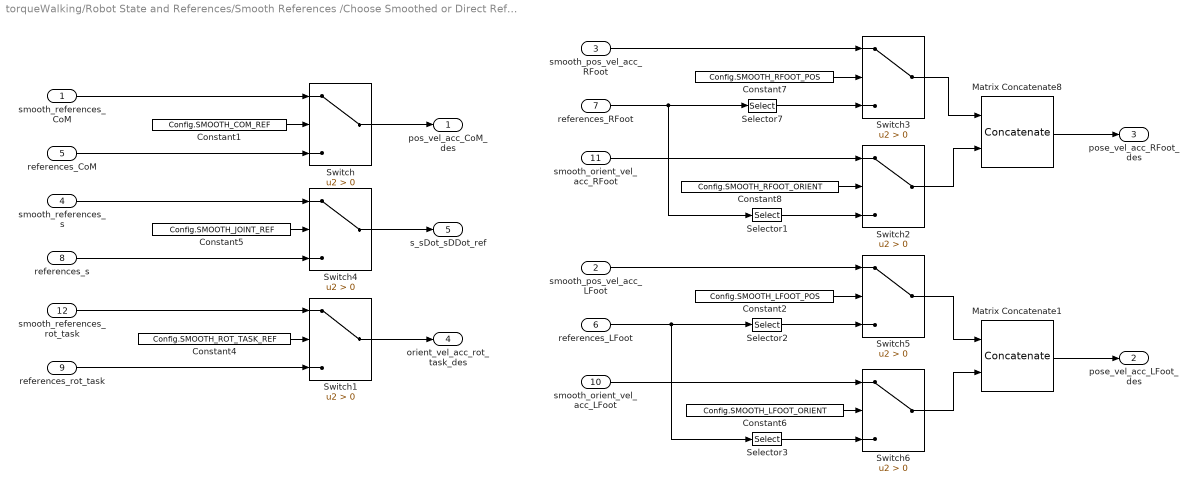
== system torqueWalking/Robot State and References/Smooth References /Choose Smoothed or Direct References ==
  smooth_references_CoM : Inport
  smooth_pos_vel_acc_LFoot : Inport  Port=2
  smooth_pos_vel_acc_RFoot : Inport  Port=3
  smooth_references_s : Inport  Port=4
  references_CoM : Inport  Port=5
  references_LFoot : Inport  Port=6
  references_RFoot : Inport  Port=7
  references_s : Inport  Port=8
  references_rot_task : Inport  Port=9
  smooth_orient_vel_acc_LFoot : Inport  Port=10
  smooth_orient_vel_acc_RFoot : Inport  Port=11
  smooth_references_rot_task : Inport  Port=12
  Constant1 : Constant  Value=Config.SMOOTH_COM_REF
  Constant2 : Constant  Value=Config.SMOOTH_LFOOT_POS
  Constant4 : Constant  Value=Config.SMOOTH_ROT_TASK_REF
  Constant5 : Constant  Value=Config.SMOOTH_JOINT_REF
  Constant6 : Constant  Value=Config.SMOOTH_LFOOT_ORIENT
  Constant7 : Constant  Value=Config.SMOOTH_RFOOT_POS
  Constant8 : Constant  Value=Config.SMOOTH_RFOOT_ORIENT
  Matrix Concatenate1 : Concatenate  Mode=Multidimensional array
  Matrix Concatenate8 : Concatenate  Mode=Multidimensional array
  Selector1 : Selector  NumberOfDimensions=2  InputPortWidth=ROBOT_DOF  IndexOptions=Index vector (dialog),Index vector (dialog)  Indices=[4:6],[1:5]  OutputSizes=1,1
  Selector2 : Selector  NumberOfDimensions=2  InputPortWidth=ROBOT_DOF  IndexOptions=Index vector (dialog),Index vector (dialog)  Indices=[1:3],[1:5]  OutputSizes=1,1
  Selector3 : Selector  NumberOfDimensions=2  InputPortWidth=ROBOT_DOF  IndexOptions=Index vector (dialog),Index vector (dialog)  Indices=[4:6],[1:5]  OutputSizes=1,1
  Selector7 : Selector  NumberOfDimensions=2  InputPortWidth=ROBOT_DOF  IndexOptions=Index vector (dialog),Index vector (dialog)  Indices=[1:3],[1:5]  OutputSizes=1,1
  Switch{,1..6} (7 alike) : Switch  Criteria=u2 > Threshold
  pos_vel_acc_CoM_des : Outport
  pose_vel_acc_LFoot_des : Outport  Port=2
  pose_vel_acc_RFoot_des : Outport  Port=3
  orient_vel_acc_rot_task_des : Outport  Port=4
  s_sDot_sDDot_ref : Outport  Port=5
  wires:
  Constant1/1 -> Switch/2
  Switch/1 -> pos_vel_acc_CoM_des/1
  Constant5/1 -> Switch4/2
  Switch4/1 -> s_sDot_sDDot_ref/1
  references_CoM/1 -> Switch/3
  smooth_references_CoM/1 -> Switch/1
  smooth_references_s/1 -> Switch4/1
  references_s/1 -> Switch4/3
  smooth_references_rot_task/1 -> Switch1/1
  references_rot_task/1 -> Switch1/3
  Constant4/1 -> Switch1/2
  Switch1/1 -> orient_vel_acc_rot_task_des/1
  smooth_pos_vel_acc_RFoot/1 -> Switch3/1
  Constant7/1 -> Switch3/2
  references_RFoot/1 -> Selector1/1, Selector7/1
  Selector7/1 -> Switch3/3
  smooth_orient_vel_acc_RFoot/1 -> Switch2/1
  Constant8/1 -> Switch2/2
  Selector1/1 -> Switch2/3
  Switch3/1 -> Matrix Concatenate8/1
  Switch2/1 -> Matrix Concatenate8/2
  references_LFoot/1 -> Selector3/1, Selector2/1
  Matrix Concatenate8/1 -> pose_vel_acc_RFoot_des/1
  Constant6/1 -> Switch6/2
  Matrix Concatenate1/1 -> pose_vel_acc_LFoot_des/1
  Switch5/1 -> Matrix Concatenate1/1
  Switch6/1 -> Matrix Concatenate1/2
  Constant2/1 -> Switch5/2
  Selector2/1 -> Switch5/3
  smooth_pos_vel_acc_LFoot/1 -> Switch5/1
  smooth_orient_vel_acc_LFoot/1 -> Switch6/1
  Selector3/1 -> Switch6/3

== system torqueWalking/Robot State and References/Smooth References /Smooth Reference Orientations ==
  w_R_LFoot_des : Inport
  w_R_RFoot_des : Inport  Port=2
  w_R_Rot_task_des : Inport  Port=3
  state : Inport  Port=4
  Compose Smoothed References : Subsystem
  Compute Ref Ang Velocities and Accelerations : Subsystem
  Compute Smoothed Ref Orientations : Subsystem
  smooth_orient_vel_acc_LFoot : Outport
  smooth_orient_vel_acc_RFoot : Outport  Port=2
  smooth_orient_vel_acc_Rot_task : Outport  Port=3
  wires:
  w_R_LFoot_des/1 -> Compute Ref Ang Velocities and Accelerations/1(w_R_LFoot_des), Compute Smoothed Ref Orientations/1(w_R_LFoot_des)
  w_R_RFoot_des/1 -> Compute Ref Ang Velocities and Accelerations/2(w_R_RFoot_des), Compute Smoothed Ref Orientations/2(w_R_RFoot_des)
  w_R_Rot_task_des/1 -> Compute Ref Ang Velocities and Accelerations/3(w_R_rot_task_des), Compute Smoothed Ref Orientations/3(w_R_rot_task_des)
  state/1 -> Compute Ref Ang Velocities and Accelerations/4(state)
  Compute Ref Ang Velocities and Accelerations/3(omega_rot_task) -> Compose Smoothed References/9(omega_rot_task), Compute Smoothed Ref Orientations/6(omega_rot_task)
  Compute Ref Ang Velocities and Accelerations/2(omega_RFoot) -> Compose Smoothed References/8(omega_RFoot), Compute Smoothed Ref Orientations/5(omega_RFoot)
  Compute Ref Ang Velocities and Accelerations/1(omega_LFoot) -> Compose Smoothed References/7(omega_LFoot), Compute Smoothed Ref Orientations/4(omega_LFoot)
  Compute Smoothed Ref Orientations/1(w_R_LFoot) -> Compose Smoothed References/6(w_R_LFoot), Compute Ref Ang Velocities and Accelerations/5(w_R_LFoot)
  Compute Smoothed Ref Orientations/2(w_R_RFoot) -> Compose Smoothed References/5(w_R_RFoot), Compute Ref Ang Velocities and Accelerations/6(w_R_RFoot)
  Compute Smoothed Ref Orientations/3(w_R_rot_task) -> Compose Smoothed References/4(w_R_rot_task), Compute Ref Ang Velocities and Accelerations/7(w_R_rot_task)
  Compute Ref Ang Velocities and Accelerations/4(omegaDot_LFoot) -> Compose Smoothed References/1(omegaDot_LFoot)
  Compute Ref Ang Velocities and Accelerations/5(omegaDot_RFoot) -> Compose Smoothed References/2(omegaDot_RFoot)
  Compute Ref Ang Velocities and Accelerations/6(omegaDot_rot_task) -> Compose Smoothed References/3(omegaDot_rot_task)
  Compose Smoothed References/1(orient_vel_acc_LFoot_des) -> smooth_orient_vel_acc_LFoot/1
  Compose Smoothed References/2(orient_vel_acc_RFoot_des) -> smooth_orient_vel_acc_RFoot/1
  Compose Smoothed References/3(orient_vel_acc_rot_task_des) -> smooth_orient_vel_acc_Rot_task/1

== system torqueWalking/Robot State and References/Smooth References /Smooth Reference Positions ==
  pos_CoM_des : Inport
  pos_LFoot_des : Inport  Port=2
  pos_RFoot_des : Inport  Port=3
  s_des : Inport  Port=4
  state : Inport  Port=5
  Configure Settling Times : MATLAB Function  TreatAsAtomicUnit=on
  Matrix Concatenate1 : Concatenate  NumInputs=3  Mode=Multidimensional array  ConcatenateDimension=2
  Matrix Concatenate2 : Concatenate  NumInputs=4  Mode=Multidimensional array  ConcatenateDimension=2
  Matrix Concatenate3 : Concatenate  NumInputs=4  Mode=Multidimensional array  ConcatenateDimension=2
  Matrix Concatenate4 : Concatenate  NumInputs=3  Mode=Multidimensional array  ConcatenateDimension=2
  Minimum Jerk Trajectory Generator{,1..3} (4 alike) : WBToolboxLibrary/Utilities/Minimum Jerk Trajectory Generator  externalSettlingTime=on  settlingTime=3  sampleTime=Config.t_step  resetOnSettlingTime=off  firstDerivatives=on  secondDerivatives=on  explicitInitialValue=off
  Settling time1 : Constant  Value=zeros(3,2)
  smooth_references_CoM : Outport
  smooth_pos_vel_acc_LFoot : Outport  Port=2
  smooth_pos_vel_acc_RFoot : Outport  Port=3
  smooth_references_s : Outport  Port=4
  wires:
  Minimum Jerk Trajectory Generator2/2 -> Matrix Concatenate3/2
  pos_LFoot_des/1 -> Minimum Jerk Trajectory Generator2/1
  pos_RFoot_des/1 -> Minimum Jerk Trajectory Generator3/1
  Minimum Jerk Trajectory Generator2/3 -> Matrix Concatenate3/3
  Minimum Jerk Trajectory Generator2/1 -> Matrix Concatenate3/1
  Minimum Jerk Trajectory Generator1/3 -> Matrix Concatenate1/3
  Matrix Concatenate1/1 -> smooth_references_s/1
  Matrix Concatenate4/1 -> smooth_references_CoM/1
  Minimum Jerk Trajectory Generator1/1 -> Matrix Concatenate1/1
  pos_CoM_des/1 -> Minimum Jerk Trajectory Generator/1
  Minimum Jerk Trajectory Generator/3 -> Matrix Concatenate4/3
  Minimum Jerk Trajectory Generator/2 -> Matrix Concatenate4/2
  Minimum Jerk Trajectory Generator1/2 -> Matrix Concatenate1/2
  Minimum Jerk Trajectory Generator3/3 -> Matrix Concatenate2/3
  Matrix Concatenate3/1 -> smooth_pos_vel_acc_LFoot/1
  Matrix Concatenate2/1 -> smooth_pos_vel_acc_RFoot/1
  Minimum Jerk Trajectory Generator/1 -> Matrix Concatenate4/1
  Minimum Jerk Trajectory Generator3/2 -> Matrix Concatenate2/2
  s_des/1 -> Minimum Jerk Trajectory Generator1/1
  Settling time1/1 -> Matrix Concatenate2/4, Matrix Concatenate3/4
  Minimum Jerk Trajectory Generator3/1 -> Matrix Concatenate2/1
  state/1 -> Configure Settling Times/1(state)
  Configure Settling Times/1(smoothingTime_CoM) -> Minimum Jerk Trajectory Generator/2
  Configure Settling Times/2(smoothingTime_LFoot) -> Minimum Jerk Trajectory Generator1/2
  Configure Settling Times/3(smoothingTime_RFoot) -> Minimum Jerk Trajectory Generator2/2
  Configure Settling Times/4(smoothingTime_joints) -> Minimum Jerk Trajectory Generator3/2

== system torqueWalking/Robot State and References/State Machines/Base to Fixed Link Transform ==
  s : Inport
  w_H_base_fixed : Inport  Port=2
  IMU port : Inport  Port=3
  qt_fixed_LFoot (walking) : Inport  Port=4
  LFoot_is_active (walking) : Inport  Port=5
  qt_fixed_RFoot (walking) : Inport  Port=6
  Compute Feet to Base Link Transforms : Subsystem
  Compute Fixed Foot to World Transform (walking) : Subsystem
  w_walking_H_LFoot : Outport
  w_walking_H_RFoot : Outport  Port=2
  w_walking_H_b : Outport  Port=3
  fixed_link_H_b : Outport  Port=4
  LFoot_H_b : Outport  Port=5
  RFoot_H_b : Outport  Port=6
  wires:
  w_H_base_fixed/1 -> Compute Feet to Base Link Transforms/1(w_H_base_fixed)
  IMU port/1 -> Compute Feet to Base Link Transforms/2(IMU port)
  s/1 -> Compute Feet to Base Link Transforms/3(s)
  qt_fixed_RFoot (walking)/1 -> Compute Fixed Foot to World Transform (walking)/3(qt_fixed_RFoot (walking))
  LFoot_is_active (walking)/1 -> Compute Fixed Foot to World Transform (walking)/2(LFoot_is_active (walking))
  qt_fixed_LFoot (walking)/1 -> Compute Fixed Foot to World Transform (walking)/1(qt_fixed_LFoot (walking))
  Compute Feet to Base Link Transforms/1(LFoot_H_b) -> LFoot_H_b/1, Compute Fixed Foot to World Transform (walking)/4(fLFoot_H_b)
  Compute Feet to Base Link Transforms/2(RFoot_H_b) -> RFoot_H_b/1, Compute Fixed Foot to World Transform (walking)/5(RFoot_H_b)
  Compute Fixed Foot to World Transform (walking)/1(w_walking_H_b) -> w_walking_H_b/1
  Compute Feet to Base Link Transforms/3(fixed_link_H_b) -> fixed_link_H_b/1
  Compute Fixed Foot to World Transform (walking)/2(w_walking_H_LFoot) -> w_walking_H_LFoot/1
  Compute Fixed Foot to World Transform (walking)/3(w_walking_H_RFoot) -> w_walking_H_RFoot/1

== system torqueWalking/Robot State and References/State Machines/Compute State Velocity ==
  s : Inport
  w_H_b : Inport  Port=2
  "feetInContact " : Inport  Port=3
  Compute Base Velocity : MATLAB Function  TreatAsAtomicUnit=on
  Feet Jacobians : Subsystem
  Get Estimate : WBToolboxLibrary/wholeBodyStates/Get Estimate  estimateType=Joints Velocity  robotName=WBT_robotName  localName=WBT_modelName  wbiFile=WBT_wbiFilename  wbiList=WBT_wbiList
  Mux : Mux  Inputs=2
  nu : Outport
  wires:
  Get Estimate/1 -> Mux/2, Compute Base Velocity/4(sDot)
  Mux/1 -> nu/1
  "feetInContact "/1 -> Compute Base Velocity/3(feetInContact)
  Compute Base Velocity/1(nu_b) -> Mux/1
  s/1 -> Feet Jacobians/1(s)
  w_H_b/1 -> Feet Jacobians/2(w_H_b)
  Feet Jacobians/1(J_LFoot) -> Compute Base Velocity/1(J_LeftFoot)
  Feet Jacobians/2(J_RFoot) -> Compute Base Velocity/2(J_RightFoot)

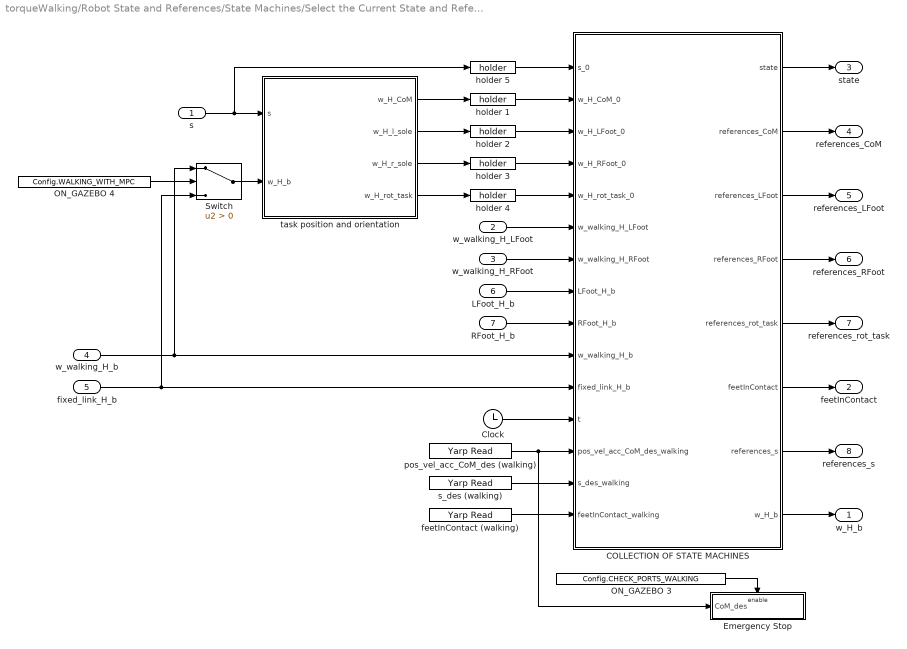
== system torqueWalking/Robot State and References/State Machines/Select the Current State and References ==
  s : Inport
  w_walking_H_LFoot : Inport  Port=2
  w_walking_H_RFoot : Inport  Port=3
  w_walking_H_b : Inport  Port=4
  fixed_link_H_b : Inport  Port=5
  LFoot_H_b : Inport  Port=6
  RFoot_H_b : Inport  Port=7
  COLLECTION OF STATE MACHINES : MATLAB Function  TreatAsAtomicUnit=on
  Clock : Clock
  Emergency Stop : Subsystem
  ON_GAZEBO 3 : Constant  Value=Config.CHECK_PORTS_WALKING
  ON_GAZEBO 4 : Constant  Value=Config.WALKING_WITH_MPC
  Switch : Switch  Criteria=u2 > Threshold
  feetInContact (walking) : WBToolboxLibrary/Utilities/Yarp Read  portName=PORTS.ACTIVE_CONTACTS  signalSize=2  blocking=off  timestamp=off  autoconnect=on  errorOnConnection=off
  holder {1..5} (5 alike) : WBToolboxLibrary/Utilities/holder 
  pos_vel_acc_CoM_des (walking) : WBToolboxLibrary/Utilities/Yarp Read  portName=PORTS.COM_DES  signalSize=9  blocking=on  timestamp=off  autoconnect=on  errorOnConnection=off
  s_des (walking) : WBToolboxLibrary/Utilities/Yarp Read  portName=PORTS.Q_DES  signalSize=15  blocking=off  timestamp=off  autoconnect=on  errorOnConnection=off
  task position and orientation : Subsystem
  w_H_b : Outport
  feetInContact : Outport  Port=2
  state : Outport  Port=3
  references_CoM : Outport  Port=4
  references_LFoot : Outport  Port=5
  references_RFoot : Outport  Port=6
  references_rot_task : Outport  Port=7
  references_s : Outport  Port=8
  wires:
  COLLECTION OF STATE MACHINES/3(references_LFoot) -> references_LFoot/1
  task position and orientation/2(w_H_l_sole) -> holder 2/1
  holder 3/1 -> COLLECTION OF STATE MACHINES/4(w_H_RFoot_0)
  COLLECTION OF STATE MACHINES/5(references_rot_task) -> references_rot_task/1
  COLLECTION OF STATE MACHINES/4(references_RFoot) -> references_RFoot/1
  s/1 -> task position and orientation/1(s), holder 5/1
  holder 4/1 -> COLLECTION OF STATE MACHINES/5(w_H_rot_task_0)
  task position and orientation/1(w_H_CoM) -> holder 1/1
  holder 2/1 -> COLLECTION OF STATE MACHINES/3(w_H_LFoot_0)
  task position and orientation/4(w_H_rot_task) -> holder 4/1
  COLLECTION OF STATE MACHINES/1(state) -> state/1
  COLLECTION OF STATE MACHINES/6(feetInContact) -> feetInContact/1
  task position and orientation/3(w_H_r_sole) -> holder 3/1
  Clock/1 -> COLLECTION OF STATE MACHINES/12(t)
  COLLECTION OF STATE MACHINES/7(references_s) -> references_s/1
  COLLECTION OF STATE MACHINES/2(references_CoM) -> references_CoM/1
  holder 1/1 -> COLLECTION OF STATE MACHINES/2(w_H_CoM_0)
  holder 5/1 -> COLLECTION OF STATE MACHINES/1(s_0)
  COLLECTION OF STATE MACHINES/8(w_H_b) -> w_H_b/1
  w_walking_H_LFoot/1 -> COLLECTION OF STATE MACHINES/6(w_walking_H_LFoot)
  w_walking_H_RFoot/1 -> COLLECTION OF STATE MACHINES/7(w_walking_H_RFoot)
  w_walking_H_b/1 -> Switch/1, COLLECTION OF STATE MACHINES/10(w_walking_H_b)
  fixed_link_H_b/1 -> Switch/3, COLLECTION OF STATE MACHINES/11(fixed_link_H_b)
  s_des (walking)/1 -> COLLECTION OF STATE MACHINES/14(s_des_walking)
  feetInContact (walking)/1 -> COLLECTION OF STATE MACHINES/15(feetInContact_walking)
  Switch/1 -> task position and orientation/2(w_H_b)
  ON_GAZEBO 4/1 -> Switch/2
  pos_vel_acc_CoM_des (walking)/1 -> COLLECTION OF STATE MACHINES/13(pos_vel_acc_CoM_des_walking), Emergency Stop/1(CoM_des)
  ON_GAZEBO 3/1 -> Emergency Stop/Enable
  LFoot_H_b/1 -> COLLECTION OF STATE MACHINES/8(LFoot_H_b)
  RFoot_H_b/1 -> COLLECTION OF STATE MACHINES/9(RFoot_H_b)

== system torqueWalking/Dynamics and Kinematics/Initial Conditions/compute state velocity/Feet Jacobians ==
  s : Inport
  w_H_b : Inport  Port=2
  Jacobian LFoot : WBToolboxLibrary/wholeBodyModel/Jacobians/Jacobian  frameName=Frames.LEFT_FOOT  robotName=WBT_robotName  localName=WBT_modelName  wbiFile=WBT_wbiFilename  wbiList=WBT_wbiList
  Jacobian RFoot : WBToolboxLibrary/wholeBodyModel/Jacobians/Jacobian  frameName=Frames.RIGHT_FOOT  robotName=WBT_robotName  localName=WBT_modelName  wbiFile=WBT_wbiFilename  wbiList=WBT_wbiList
  J_LFoot : Outport
  J_RFoot : Outport  Port=2
  wires:
  Jacobian LFoot/1 -> J_LFoot/1
  Jacobian RFoot/1 -> J_RFoot/1
  w_H_b/1 -> Jacobian RFoot/1, Jacobian LFoot/1
  s/1 -> Jacobian LFoot/2, Jacobian RFoot/2

== system torqueWalking/Dynamics and Kinematics/Inverse Kinematics/ComputeTasksPoseAndVelocity/Task position and orientation ==
  s : Inport
  w_H_b : Inport  Port=2
  CoM : WBToolboxLibrary/wholeBodyModel/Kinematics/Forward Kinematics  frameName=Frames.COM  robotName=WBT_robotName  localName=WBT_modelName  wbiFile=WBT_wbiFilename  wbiList=WBT_wbiList
  LFoot : WBToolboxLibrary/wholeBodyModel/Kinematics/Forward Kinematics  frameName=Frames.LEFT_FOOT  robotName=WBT_robotName  localName=WBT_modelName  wbiFile=WBT_wbiFilename  wbiList=WBT_wbiList
  RFoot : WBToolboxLibrary/wholeBodyModel/Kinematics/Forward Kinematics  frameName=Frames.RIGHT_FOOT  robotName=WBT_robotName  localName=WBT_modelName  wbiFile=WBT_wbiFilename  wbiList=WBT_wbiList
  rotational task : WBToolboxLibrary/wholeBodyModel/Kinematics/Forward Kinematics  frameName=Frames.ROT_TASK_LINK  robotName=WBT_robotName  localName=WBT_modelName  wbiFile=WBT_wbiFilename  wbiList=WBT_wbiList
  w_H_CoM : Outport
  w_H_l_sole : Outport  Port=2
  w_H_r_sole : Outport  Port=3
  w_H_rot_task : Outport  Port=4
  wires:
  s/1 -> rotational task/2, RFoot/2, LFoot/2, CoM/2
  w_H_b/1 -> rotational task/1, CoM/1, LFoot/1, RFoot/1
  CoM/1 -> w_H_CoM/1
  LFoot/1 -> w_H_l_sole/1
  RFoot/1 -> w_H_r_sole/1
  rotational task/1 -> w_H_rot_task/1

== system torqueWalking/Dynamics and Kinematics/Inverse Kinematics/QP-Based Inverse Kinematics/QP Solver (inverse kinematics) ==
  Hessian : Inport
  gradient : Inport  Port=2
  ConstraintMatrix : Inport  Port=3
  biasVectorConstraint : Inport  Port=4
  QPSolver : M-S-Function  FunctionName=QPInverseKinematics  Parameters=ROBOT_DOF, Sat, Config
  nuDot : Outport
  ExitFlagQP : Outport  Port=2
  wires:
  QPSolver/1 -> nuDot/1
  QPSolver/2 -> ExitFlagQP/1
  Hessian/1 -> QPSolver/1
  gradient/1 -> QPSolver/2
  biasVectorConstraint/1 -> QPSolver/4
  ConstraintMatrix/1 -> QPSolver/3
